simulink model "E_a_b_Idealna_Realna_staticka_karakteristika"  (R2016a)
settings: Solver=VariableStepAuto  StartTime=0.0  StopTime=100  RelTol=1e-3
libraries: simulink x1
settings Model: Creator=AmelT  LastModifiedBy=AmelT

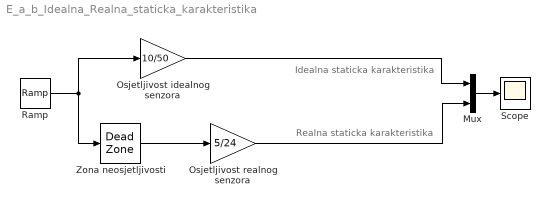
== system E_a_b_Idealna_Realna_staticka_karakteristika ==
  note: Realna staticka karakteristika
  note: Idealna staticka karakteristika
  Mux : Mux  Inputs=2
  Osjetljivost idealnog senzora : Gain  Gain=10/50
  Osjetljivost realnog senzora : Gain  Gain=5/24
  Ramp : simulink/Sources/Ramp  slope=1  start=0  X0=-50
  Scope : Scope
  Zona neosjetljivosti : DeadZone  LowerValue=-2  UpperValue=2  SaturateOnIntegerOverflow=on
  wires:
  Ramp/1 -> Osjetljivost idealnog senzora/1, Zona neosjetljivosti/1
  Zona neosjetljivosti/1 -> Osjetljivost realnog senzora/1
  Osjetljivost realnog senzora/1 -> Mux/2
  Osjetljivost idealnog senzora/1 -> Mux/1
  Mux/1 -> Scope/1
